simulink model "thermal_model_of_IGBT_module"  (R2015a)
settings: Solver=ode1  StartTime=0.0  StopTime=10.0  FixedStep=10  RelTol=1e-3
settings Model: Creator=Caner  LastModifiedBy=Caner

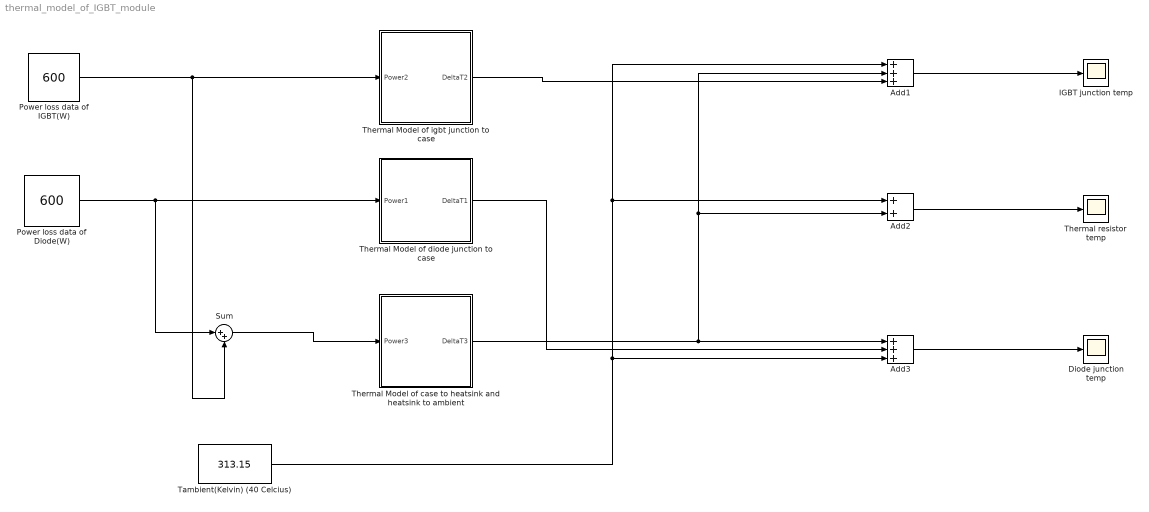
== system thermal_model_of_IGBT_module ==
  Add1 : Sum  Inputs=+++
  Add2 : Sum
  Add3 : Sum  Inputs=+++
  Diode junction temp : Scope
  IGBT junction temp : Scope
  "Power loss data of Diode(W) " : Constant  Value=600  SampleTime=10
  Power loss data of IGBT(W) : Constant  Value=600  SampleTime=10
  Sum : Sum  Inputs=|++
  Tambient(Kelvin) (40 Celcius) : Constant  Value=313.15
  Thermal Model of case to heatsink and heatsink to ambient : Subsystem
  Thermal Model of diode junction to case : Subsystem
  Thermal Model of igbt junction to case : Subsystem
  Thermal resistor temp : Scope
      settings: SaveName=ScopeData2
  wires:
  Power loss data of IGBT(W)/1 -> Thermal Model of igbt junction to case/1(Power2), Sum/2
  "Power loss data of Diode(W) "/1 -> Sum/1, Thermal Model of diode junction to case/1(Power1)
  Sum/1 -> Thermal Model of case to heatsink and heatsink to ambient/1(Power3)
  Thermal Model of case to heatsink and heatsink to ambient/1(DeltaT3) -> Add3/1, Add1/2, Add2/2
  Tambient(Kelvin) (40 Celcius)/1 -> Add3/3, Add1/1, Add2/1
  Add1/1 -> IGBT junction temp/1
  Add2/1 -> Thermal resistor temp/1
  Add3/1 -> Diode junction temp/1
  Thermal Model of diode junction to case/1(DeltaT1) -> Add3/2
  Thermal Model of igbt junction to case/1(DeltaT2) -> Add1/3

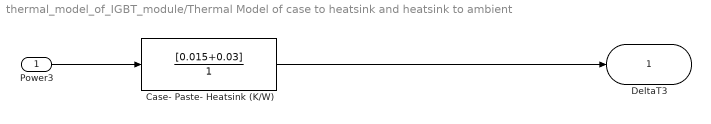
== system thermal_model_of_IGBT_module/Thermal Model of case to heatsink and heatsink to ambient ==
  Power3 : Inport
  Case- Paste- Heatsink (K/W) : DiscreteTransferFcn  Numerator=[0.015+0.03]  Denominator=[1]
  DeltaT3 : Outport
  wires:
  Case- Paste- Heatsink (K/W)/1 -> DeltaT3/1
  Power3/1 -> Case- Paste- Heatsink (K/W)/1

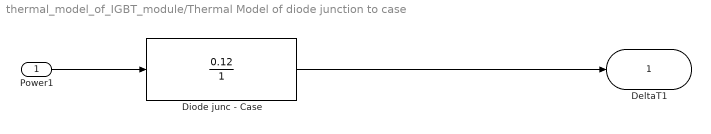
== system thermal_model_of_IGBT_module/Thermal Model of diode junction to case ==
  Power1 : Inport
  Diode junc - Case : DiscreteTransferFcn  Numerator=[0.12]  Denominator=[1]
  DeltaT1 : Outport
  wires:
  Diode junc - Case/1 -> DeltaT1/1
  Power1/1 -> Diode junc - Case/1

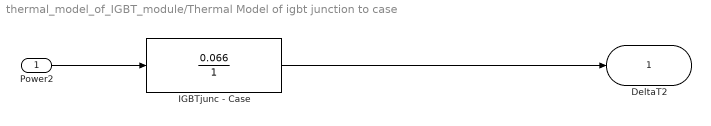
== system thermal_model_of_IGBT_module/Thermal Model of igbt junction to case ==
  Power2 : Inport
  IGBTjunc - Case : DiscreteTransferFcn  Numerator=[0.066]  Denominator=[1]
  DeltaT2 : Outport
  wires:
  IGBTjunc - Case/1 -> DeltaT2/1
  Power2/1 -> IGBTjunc - Case/1
